simulink model "softMBD_old"  (R2025b)
settings: Solver=FixedStepAuto  StartTime=0.0  StopTime=10  FixedStep=0.005  RelTol=1e-3
values from neighbouring files (symbols this model uses):
  FPV_mass = 0.8    [Soft.m]
  g = 9.81    [Soft.m]
  ks = 0    [Soft.m]
  p_0 = 1013.25    [Soft.m]
  Q2Ts = forcetomotors()    [Soft.m]    (also in forcetomotors.m = inv(Ts2Q))
  takeOffDuration = 2    [Soft.m]
  Ts = 0.005    [Soft.m]
undefined symbols (not defined in the file or in its folder): DiscIntNeverNeededParam, kd_pq, kd_pr, kd_y, ki_pq, ki_pr, ki_t, ki_y, kp_pq, kp_pr, kp_y, pInitialization
libraries: simulink x35, discretizing x11, slpidlib x2, shared6dof x1, dynamicsLibrary x1, aerolibasang x1, aerolibnav x1
(part 17 of 20)

== system softMBD_old/FCS/Controller/roll_pitch_controller/PID Controller/Saturation Fdbk/Enabled ==
  In1 : Inport  SampleTime=SampleTime
  Saturation : Saturate  UpperLimit=UpperSaturationLimit  LowerLimit=LowerSaturationLimit  SampleTime=SampleTime  OutMin=SaturationOutMin  OutMax=SaturationOutMax
  Out1 : Outport  SampleTime=SampleTime
  wires:
  Saturation/1 -> Out1/1
  In1/1 -> Saturation/1

== system softMBD_old/FCS/Controller/roll_pitch_controller/PID Controller/Saturation Fdbk/External ==
  In1 : Inport  SampleTime=SampleTime
  Upper Limit : Inport  Port=2  SampleTime=SampleTime
  Lower Limit : Inport  Port=3  SampleTime=SampleTime
  Saturation Dynamic : simulink/Discontinuities/Saturation Dynamic  OutMin=SaturationOutMin  OutMax=SaturationOutMax  OutDataTypeStr=Inherit: Same as second input  OutDataType=fixdt(1, 16)  OutScaling=2^-10  DoSatur=off
  Out1 : Outport  SampleTime=SampleTime
  wires:
  Lower Limit/1 -> Saturation Dynamic/3
  Upper Limit/1 -> Saturation Dynamic/1
  Saturation Dynamic/1 -> Out1/1
  In1/1 -> Saturation Dynamic/2

== system softMBD_old/FCS/Controller/roll_pitch_controller/PID Controller/Saturation Fdbk/Passthrough ==
  In1 : Inport  SampleTime=SampleTime
  Out1 : Outport  SampleTime=SampleTime
  wires:
  In1/1 -> Out1/1

== system softMBD_old/FCS/Controller/roll_pitch_controller/PID Controller/Sum/Passthrough_I ==
  P : Inport  SampleTime=SampleTime
  I : Inport  Port=2  SampleTime=SampleTime
  Signal Specification : SignalSpecification  OutDataTypeStr=boolean  SampleTime=SampleTime
  Terminator : Terminator
  Out1 : Outport  SampleTime=SampleTime
  wires:
  Signal Specification/1 -> Terminator/1
  P/1 -> Signal Specification/1
  I/1 -> Out1/1

== system softMBD_old/FCS/Controller/roll_pitch_controller/PID Controller/Sum/Passthrough_P ==
  P : Inport  SampleTime=SampleTime
  Out1 : Outport  SampleTime=SampleTime
  wires:
  P/1 -> Out1/1

== system softMBD_old/FCS/Controller/roll_pitch_controller/PID Controller/Sum/Sum_PD ==
  P : Inport  SampleTime=SampleTime
  D : Inport  Port=2  SampleTime=SampleTime
  Sum : Sum  Inputs=|++  OutMin=SumOutMin  OutMax=SumOutMax
  Out1 : Outport  SampleTime=SampleTime
  wires:
  P/1 -> Sum/1
  D/1 -> Sum/2
  Sum/1 -> Out1/1

== system softMBD_old/FCS/Controller/roll_pitch_controller/PID Controller/Sum/Sum_PI ==
  P : Inport  SampleTime=SampleTime
  I : Inport  Port=2  SampleTime=SampleTime
  Sum : Sum  Inputs=|++  OutMin=SumOutMin  OutMax=SumOutMax
  Out1 : Outport  SampleTime=SampleTime
  wires:
  I/1 -> Sum/2
  P/1 -> Sum/1
  Sum/1 -> Out1/1

== system softMBD_old/FCS/Controller/roll_pitch_controller/PID Controller/Sum/Sum_PID ==
  P : Inport  SampleTime=SampleTime
  I : Inport  Port=2  SampleTime=SampleTime
  D : Inport  Port=3  SampleTime=SampleTime
  Sum : Sum  Inputs=+++  OutMin=SumOutMin  OutMax=SumOutMax
  Out1 : Outport  SampleTime=SampleTime
  wires:
  I/1 -> Sum/2
  P/1 -> Sum/1
  D/1 -> Sum/3
  Sum/1 -> Out1/1

== system softMBD_old/FCS/Controller/roll_pitch_controller/PID Controller/Sum Fdbk/Disabled ==
  fromP : Inport  SampleTime=SampleTime
  fromState : Inport  Port=2  SampleTime=SampleTime
  fromD : Inport  Port=3  SampleTime=SampleTime
  Signal Specification1 : SignalSpecification  DisableCoverage=on  OutDataTypeStr=boolean  SampleTime=SampleTime
  Terminator1 : Terminator
  Terminator2 : Terminator
  Terminator3 : Terminator
  wires:
  fromD/1 -> Terminator3/1
  fromState/1 -> Signal Specification1/1
  fromP/1 -> Terminator1/1
  Signal Specification1/1 -> Terminator2/1

== system softMBD_old/FCS/Controller/roll_pitch_controller/PID Controller/Sum Fdbk/Enabled ==
  fromP : Inport  SampleTime=SampleTime
  fromState : Inport  Port=2  SampleTime=SampleTime
  fromD : Inport  Port=3  SampleTime=SampleTime
  Sum Fdbk : Sum  DisableCoverage=on  Inputs=+++  OutMin=SumOutMin  OutMax=SumOutMax
  Out1 : Outport  SampleTime=SampleTime
  wires:
  fromP/1 -> Sum Fdbk/1
  fromState/1 -> Sum Fdbk/2
  fromD/1 -> Sum Fdbk/3
  Sum Fdbk/1 -> Out1/1

== system softMBD_old/FCS/Controller/roll_pitch_controller/PID Controller/Sum Fdbk/Passthrough ==
  fromState : Inport  SampleTime=SampleTime
  Out1 : Outport  SampleTime=SampleTime
  wires:
  fromState/1 -> Out1/1

== system softMBD_old/FCS/Controller/roll_pitch_controller/PID Controller/Tracking Mode/Disabled ==
  uout : Inport  SampleTime=SampleTime
  TR : Inport  Port=2  SampleTime=SampleTime
  Signal Specification1 : SignalSpecification  DisableCoverage=on  OutDataTypeStr=boolean  SampleTime=SampleTime
  Terminator1 : Terminator
  Terminator3 : Terminator
  wires:
  uout/1 -> Terminator3/1
  TR/1 -> Signal Specification1/1
  Signal Specification1/1 -> Terminator1/1

== system softMBD_old/FCS/Controller/roll_pitch_controller/PID Controller/Tracking Mode/Enabled ==
  uout : Inport  SampleTime=SampleTime
  TR : Inport  Port=2  SampleTime=SampleTime
  Kt : Gain  Gain=Kt  ParamMin=KtParamMin  ParamMax=KtParamMax  OutMin=KtOutMin  OutMax=KtOutMax
  SumI3 : Sum  Inputs=|-+  OutMin=SumI3OutMin  OutMax=SumI3OutMax
  Out1 : Outport  SampleTime=SampleTime
  wires:
  Kt/1 -> Out1/1
  SumI3/1 -> Kt/1
  TR/1 -> SumI3/2
  uout/1 -> SumI3/1

== system softMBD_old/FCS/Controller/roll_pitch_controller/PID Controller/Tracking Mode Sum/Passthrough ==
  fromIgain : Inport  SampleTime=SampleTime
  fromTR : Inport  Port=2  SampleTime=SampleTime
  Signal Specification : SignalSpecification  DisableCoverage=on  OutDataTypeStr=boolean  SampleTime=SampleTime
  Terminator : Terminator
  preInt : Outport
  wires:
  fromIgain/1 -> preInt/1
  fromTR/1 -> Signal Specification/1
  Signal Specification/1 -> Terminator/1

== system softMBD_old/FCS/Controller/roll_pitch_controller/PID Controller/Tracking Mode Sum/Tracking Mode ==
  fromIgain : Inport  SampleTime=SampleTime
  fromTR : Inport  Port=2  SampleTime=SampleTime
  SumI1 : Sum  Inputs=|++  OutMin=SumI1OutMin  OutMax=SumI1OutMax
  preInt : Outport
  wires:
  fromIgain/1 -> SumI1/1
  fromTR/1 -> SumI1/2
  SumI1/1 -> preInt/1

== system softMBD_old/FCS/Controller/roll_pitch_controller/PID Controller/Tsamp - Integral/Disabled ==
  U : Inport  SampleTime=SampleTime
  Ts : Inport  Port=2  SampleTime=SampleTime
  Terminator : Terminator
  Out1 : Outport  SampleTime=SampleTime
  wires:
  U/1 -> Out1/1
  Ts/1 -> Terminator/1

== system softMBD_old/FCS/Controller/roll_pitch_controller/PID Controller/Tsamp - Integral/External Ts ==
  U : Inport  SampleTime=SampleTime
  Ts : Inport  Port=2  SampleTime=SampleTime
  Uintegral*Ts Prod Out : Product  OutMin=UintegralTsProdOutMin  OutMax=UintegralTsProdOutMax  SampleTime=SampleTime
  Out1 : Outport  SampleTime=SampleTime
  wires:
  U/1 -> Uintegral*Ts Prod Out/1
  Uintegral*Ts Prod Out/1 -> Out1/1
  Ts/1 -> Uintegral*Ts Prod Out/2

== system softMBD_old/FCS/Controller/roll_pitch_controller/PID Controller/Tsamp - Integral/Passthrough ==
  U : Inport  SampleTime=SampleTime
  Ts : Inport  Port=2  SampleTime=SampleTime
  Terminator : Terminator
  Out1 : Outport  SampleTime=SampleTime
  wires:
  Ts/1 -> Terminator/1
  U/1 -> Out1/1

== system softMBD_old/FCS/Controller/roll_pitch_controller/PID Controller/Tsamp - Integral/TsSignalSpecification ==
  U : Inport  SampleTime=SampleTime
  Ts : Inport  Port=2  SampleTime=SampleTime
  Signal Specification : SignalSpecification  DisableCoverage=on  OutDataTypeStr=boolean  SampleTime=SampleTime
  Terminator : Terminator
  Out1 : Outport  SampleTime=SampleTime
  wires:
  U/1 -> Out1/1
  Ts/1 -> Signal Specification/1
  Signal Specification/1 -> Terminator/1

== system softMBD_old/FCS/Controller/roll_pitch_controller/PID Controller/Tsamp - Ngain/External Ts ==
  U : Inport  SampleTime=SampleTime
  Ts : Inport  Port=2  SampleTime=SampleTime
  Ungain*Ts Prod Out : Product  OutMin=UngainTsProdOutMin  OutMax=UngainTsProdOutMax  SampleTime=SampleTime
  Out1 : Outport  SampleTime=SampleTime
  wires:
  Ts/1 -> Ungain*Ts Prod Out/2
  Ungain*Ts Prod Out/1 -> Out1/1
  U/1 -> Ungain*Ts Prod Out/1

== system softMBD_old/FCS/Controller/roll_pitch_controller/PID Controller/Tsamp - Ngain/Passthrough ==
  U : Inport  SampleTime=SampleTime
  Ts : Inport  Port=2  SampleTime=SampleTime
  Terminator : Terminator
  Out1 : Outport  SampleTime=SampleTime
  wires:
  U/1 -> Out1/1
  Ts/1 -> Terminator/1

== system softMBD_old/FCS/Controller/roll_pitch_controller/PID Controller/postSat Signal/Feedback_Path ==
  feedback : Inport  SampleTime=SampleTime
  forward : Inport  Port=2  SampleTime=SampleTime
  Terminator1 : Terminator
  Out1 : Outport  SampleTime=SampleTime
  wires:
  feedback/1 -> Out1/1
  forward/1 -> Terminator1/1

== system softMBD_old/FCS/Controller/roll_pitch_controller/PID Controller/postSat Signal/Forward_Path ==
  feedback : Inport  SampleTime=SampleTime
  forward : Inport  Port=2  SampleTime=SampleTime
  Signal Specification1 : SignalSpecification  DisableCoverage=on  OutDataTypeStr=boolean  SampleTime=SampleTime
  Terminator1 : Terminator
  Out1 : Outport  SampleTime=SampleTime
  wires:
  forward/1 -> Out1/1
  feedback/1 -> Signal Specification1/1
  Signal Specification1/1 -> Terminator1/1

== system softMBD_old/FCS/Controller/roll_pitch_controller/PID Controller/preInt Signal/External PreInt ==
  preInt : Inport  SampleTime=SampleTime
  extAW : Inport  Port=2  SampleTime=SampleTime
  Terminator1 : Terminator
  Out1 : Outport  SampleTime=SampleTime
  wires:
  preInt/1 -> Terminator1/1
  extAW/1 -> Out1/1

== system softMBD_old/FCS/Controller/roll_pitch_controller/PID Controller/preInt Signal/Internal PreInt ==
  preInt : Inport  SampleTime=SampleTime
  extAW : Inport  Port=2  SampleTime=SampleTime
  Signal Specification1 : SignalSpecification  DisableCoverage=on  OutDataTypeStr=boolean  SampleTime=SampleTime
  Terminator1 : Terminator
  Out1 : Outport  SampleTime=SampleTime
  wires:
  Signal Specification1/1 -> Terminator1/1
  extAW/1 -> Signal Specification1/1
  preInt/1 -> Out1/1

== system softMBD_old/FCS/Controller/roll_pitch_controller/PID Controller/preSat Signal/Feedback_Path ==
  feedback : Inport  SampleTime=SampleTime
  forward : Inport  Port=2  SampleTime=SampleTime
  Terminator1 : Terminator
  Out1 : Outport  SampleTime=SampleTime
  wires:
  feedback/1 -> Out1/1
  forward/1 -> Terminator1/1

== system softMBD_old/FCS/Controller/roll_pitch_controller/PID Controller/preSat Signal/Forward_Path ==
  feedback : Inport  SampleTime=SampleTime
  forward : Inport  Port=2  SampleTime=SampleTime
  Signal Specification1 : SignalSpecification  DisableCoverage=on  OutDataTypeStr=boolean  SampleTime=SampleTime
  Terminator1 : Terminator
  Out1 : Outport  SampleTime=SampleTime
  wires:
  forward/1 -> Out1/1
  feedback/1 -> Signal Specification1/1
  Signal Specification1/1 -> Terminator1/1

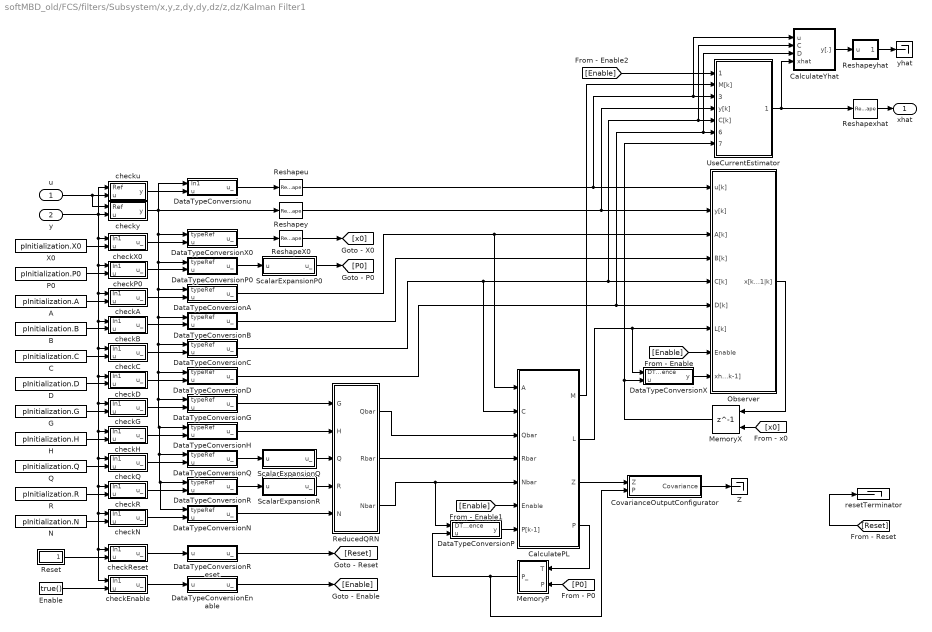
== system softMBD_old/FCS/filters/Subsystem/x,y,z,dy,dy,dz/z,dz/Kalman Filter1 ==
  u : Inport
  y : Inport  Port=2
  A : Constant  Value=pInitialization.A  VectorParams1D=off  OutDataTypeStr=Inherit: Inherit via back propagation
  B : Constant  Value=pInitialization.B  VectorParams1D=off  OutDataTypeStr=Inherit: Inherit via back propagation
  C : Constant  Value=pInitialization.C  VectorParams1D=off  OutDataTypeStr=Inherit: Inherit via back propagation
  CalculatePL : Subsystem  AncestorBlock=ctrlSharedLib/KalmanFilterUtilities/ConstantPL  mask(ctrlKalmanFilterConstantPL){}
  CalculateYhat : Subsystem  AncestorBlock=ctrlSharedLib/KalmanFilterUtilities/DontCalculateYhat  mask(ctrlKalmanFilterDontCalculateYhat){}
  CovarianceOutputConfigurator : Subsystem
  D : Constant  Value=pInitialization.D  VectorParams1D=off  OutDataTypeStr=Inherit: Inherit via back propagation
  DataTypeConversionA : Subsystem  AncestorBlock=ctrlSharedLib/Utilities/DataTypeDuplicateAndOutput  mask(ctrlDataTypeDuplicateAndOutput){}
  DataTypeConversionB : Subsystem  AncestorBlock=ctrlSharedLib/Utilities/DataTypeDuplicateAndOutput  mask(ctrlDataTypeDuplicateAndOutput){}
  DataTypeConversionC : Subsystem  AncestorBlock=ctrlSharedLib/Utilities/DataTypeDuplicateAndOutput  mask(ctrlDataTypeDuplicateAndOutput){}
  DataTypeConversionD : Subsystem  AncestorBlock=ctrlSharedLib/Utilities/DataTypeDuplicateAndOutput  mask(ctrlDataTypeDuplicateAndOutput){}
  DataTypeConversionEnable : Subsystem  AncestorBlock=ctrlSharedLib/Utilities/PassInputThrough
  DataTypeConversionG : Subsystem  AncestorBlock=ctrlSharedLib/Utilities/DataTypeDuplicateAndOutput  mask(ctrlDataTypeDuplicateAndOutput){}
  DataTypeConversionH : Subsystem  AncestorBlock=ctrlSharedLib/Utilities/DataTypeDuplicateAndOutput  mask(ctrlDataTypeDuplicateAndOutput){}
  DataTypeConversionN : Subsystem  AncestorBlock=ctrlSharedLib/Utilities/DataTypeDuplicateAndOutput  mask(ctrlDataTypeDuplicateAndOutput){}
  DataTypeConversionP : Subsystem  AncestorBlock=|  mask(Conversion Inherited){ConvertRealWorld=Real World Value, RndMeth=Floor, DoSatur=off}
      | simulink/Signal
      | Attributes/Data Type
      | Conversion
      | Inherited
      mask prompts: ConvertRealWorld "Simulink:masks:InputAndOutputToHaveEqual_MP"; RndMeth "Simulink:masks:IntegerRoundingMode_MP"; DoSatur "Simulink:masks:SaturateToMaxOrMinWhenOverflowsOccur_MP"
      mask help: Simulink:masks:ConversionInherited_MD
      mask init: same as softMBD_old/FCS/filters/Subsystem1/pitch_kalman/Kalman Filter1/DataTypeConversionP
      mask TypeOptions ConvertRealWorld: Simulink:masks:RealWorldValue | Simulink:masks:StoredInteger
      mask TypeOptions RndMeth: Simulink:masks:Ceiling | Simulink:masks:Convergent | Simulink:masks:Floor | Simulink:masks:Nearest | Simulink:masks:Round | Simulink:masks:Simplest | Simulink:masks:Zero
      mask Display:
      | port_label('Input',2,'u');
      | port_label('Output',1,'y');
      |     if(get_param(gcbh,'ConvertRealWorld') == "Stored Integer")
      |        disp('SI')
      |     else
      |        disp('Convert')
      |     end
  DataTypeConversionP0 : Subsystem  AncestorBlock=ctrlSharedLib/Utilities/DataTypeDuplicateAndOutput  mask(ctrlDataTypeDuplicateAndOutput){}
  DataTypeConversionQ : Subsystem  AncestorBlock=ctrlSharedLib/Utilities/DataTypeDuplicateAndOutput  mask(ctrlDataTypeDuplicateAndOutput){}
  DataTypeConversionR : Subsystem  AncestorBlock=ctrlSharedLib/Utilities/DataTypeDuplicateAndOutput  mask(ctrlDataTypeDuplicateAndOutput){}
  DataTypeConversionReset : Subsystem  AncestorBlock=ctrlSharedLib/Utilities/PassInputThrough
  DataTypeConversionX : Subsystem  AncestorBlock=|  mask(Conversion Inherited){ConvertRealWorld=Real World Value, RndMeth=Floor, DoSatur=off}
      | simulink/Signal
      | Attributes/Data Type
      | Conversion
      | Inherited
      mask prompts: ConvertRealWorld "Simulink:masks:InputAndOutputToHaveEqual_MP"; RndMeth "Simulink:masks:IntegerRoundingMode_MP"; DoSatur "Simulink:masks:SaturateToMaxOrMinWhenOverflowsOccur_MP"
      mask help: Simulink:masks:ConversionInherited_MD
      mask init: same as softMBD_old/FCS/filters/Subsystem1/pitch_kalman/Kalman Filter1/DataTypeConversionP
      mask TypeOptions ConvertRealWorld: Simulink:masks:RealWorldValue | Simulink:masks:StoredInteger
      mask TypeOptions RndMeth: Simulink:masks:Ceiling | Simulink:masks:Convergent | Simulink:masks:Floor | Simulink:masks:Nearest | Simulink:masks:Round | Simulink:masks:Simplest | Simulink:masks:Zero
      mask Display:
      | port_label('Input',2,'u');
      | port_label('Output',1,'y');
      |     if(get_param(gcbh,'ConvertRealWorld') == "Stored Integer")
      |        disp('SI')
      |     else
      |        disp('Convert')
      |     end
  DataTypeConversionX0 : Subsystem  AncestorBlock=ctrlSharedLib/Utilities/DataTypeDuplicateAndOutput  mask(ctrlDataTypeDuplicateAndOutput){}
  DataTypeConversionu : Subsystem  AncestorBlock=ctrlSharedLib/KalmanFilterUtilities/PassSecondInputThrough  mask(ctrlKalmanFilterPassSecondInputThrough){}
      mask Display:
      | port_label('Input',2,'u');
      | port_label('Output',1,'y');
  Enable : Constant  Value=true()  OutDataTypeStr=boolean
  G : Constant  Value=pInitialization.G  VectorParams1D=off  OutDataTypeStr=Inherit: Inherit via back propagation
  H : Constant  Value=pInitialization.H  VectorParams1D=off  OutDataTypeStr=Inherit: Inherit via back propagation
  MemoryP : Subsystem  AncestorBlock=ctrlSharedLib/KalmanFilterUtilities/MemoryP  mask(ctrlKalmanFilterNoMemoryP){}
      mask Display:
      | port_label('Input',2,'P');
      | port_label('Output',1,'P');
  MemoryX : Delay  DelayLength=1  InitialConditionSource=Input port  SampleTime=pInitialization.Ts
      settings: InputPortMap=u0,p4
  N : Constant  Value=pInitialization.N  VectorParams1D=off  OutDataTypeStr=Inherit: Inherit via back propagation
  Observer : Subsystem
  P0 : Constant  Value=pInitialization.P0  OutDataTypeStr=Inherit: Inherit via back propagation
  Q : Constant  Value=pInitialization.Q  VectorParams1D=off  OutDataTypeStr=Inherit: Inherit via back propagation
  R : Constant  Value=pInitialization.R  VectorParams1D=off  OutDataTypeStr=Inherit: Inherit via back propagation
  ReducedQRN : Subsystem  AncestorBlock=ctrlSharedLib/KalmanFilterUtilities/NoReducedQRN  mask(ctrlKalmanFilterNoReducedQRN){}
  Reset : Subsystem  AncestorBlock=ctrlSharedLib/Utilities/Ground  mask(ctrlSharedLibGround){OutDataTypeStr=boolean, Dimensions=1}
      mask prompts: OutDataTypeStr "Simulink:blkprm_prompts:UNIFIEDDATATYPE"; Dimensions "Simulink:blkprm_prompts:SigSpecDims"
      mask TypeOptions OutDataTypeStr: Signal Specification/OutDataTypeStr
      mask TypeOptions Dimensions: Signal Specification/Dimensions
      mask DialogControl OutDataTypeStr Prompt: Data type:
      mask DialogControl Dimensions Prompt: Dimensions (-1 for inherited):
  ReshapeX0 : Reshape
  Reshapeu : Reshape
  Reshapexhat : Reshape
  Reshapey : Reshape
  Reshapeyhat : Subsystem  AncestorBlock=ctrlSharedLib/Utilities/PassInputThrough
  ScalarExpansionP0 : Subsystem  AncestorBlock=ctrlSharedLib/Utilities/PassInputThrough
  ScalarExpansionQ : Subsystem  AncestorBlock=ctrlSharedLib/Utilities/PassInputThrough
  ScalarExpansionR : Subsystem  AncestorBlock=ctrlSharedLib/Utilities/PassInputThrough
  UseCurrentEstimator : Subsystem  AncestorBlock=ctrlSharedLib/KalmanFilterUtilities/UseCurrentEstimatorZeroD  mask(ctrlKalmanFilterUseCurrentEstimatorZeroD){}
  X0 : Constant  Value=pInitialization.X0  VectorParams1D=off  OutDataTypeStr=Inherit: Inherit via back propagation
  Z : Terminator
  checkA : Subsystem  AncestorBlock=ctrlSharedLib/KalmanFilterUtilities/PassSecondInputThrough  mask(ctrlKalmanFilterPassSecondInputThrough){}
      mask Display:
      | port_label('Input',2,'u');
      | port_label('Output',1,'y');
  checkB : Subsystem  AncestorBlock=ctrlSharedLib/KalmanFilterUtilities/PassSecondInputThrough  mask(ctrlKalmanFilterPassSecondInputThrough){}
      mask Display:
      | port_label('Input',2,'u');
      | port_label('Output',1,'y');
  checkC : Subsystem  AncestorBlock=ctrlSharedLib/KalmanFilterUtilities/PassSecondInputThrough  mask(ctrlKalmanFilterPassSecondInputThrough){}
      mask Display:
      | port_label('Input',2,'u');
      | port_label('Output',1,'y');
  checkD : Subsystem  AncestorBlock=ctrlSharedLib/KalmanFilterUtilities/PassSecondInputThrough  mask(ctrlKalmanFilterPassSecondInputThrough){}
      mask Display:
      | port_label('Input',2,'u');
      | port_label('Output',1,'y');
  checkEnable : Subsystem  AncestorBlock=ctrlSharedLib/KalmanFilterUtilities/PassSecondInputThrough  mask(ctrlKalmanFilterPassSecondInputThrough){}
      mask Display:
      | port_label('Input',2,'u');
      | port_label('Output',1,'y');
  checkG : Subsystem  AncestorBlock=ctrlSharedLib/KalmanFilterUtilities/PassSecondInputThrough  mask(ctrlKalmanFilterPassSecondInputThrough){}
      mask Display:
      | port_label('Input',2,'u');
      | port_label('Output',1,'y');
  checkH : Subsystem  AncestorBlock=ctrlSharedLib/KalmanFilterUtilities/PassSecondInputThrough  mask(ctrlKalmanFilterPassSecondInputThrough){}
      mask Display:
      | port_label('Input',2,'u');
      | port_label('Output',1,'y');
  checkN : Subsystem  AncestorBlock=ctrlSharedLib/KalmanFilterUtilities/PassSecondInputThrough  mask(ctrlKalmanFilterPassSecondInputThrough){}
      mask Display:
      | port_label('Input',2,'u');
      | port_label('Output',1,'y');
  checkP0 : Subsystem  AncestorBlock=ctrlSharedLib/KalmanFilterUtilities/PassSecondInputThrough  mask(ctrlKalmanFilterPassSecondInputThrough){}
      mask Display:
      | port_label('Input',2,'u');
      | port_label('Output',1,'y');
  checkQ : Subsystem  AncestorBlock=ctrlSharedLib/KalmanFilterUtilities/PassSecondInputThrough  mask(ctrlKalmanFilterPassSecondInputThrough){}
      mask Display:
      | port_label('Input',2,'u');
      | port_label('Output',1,'y');
  checkR : Subsystem  AncestorBlock=ctrlSharedLib/KalmanFilterUtilities/PassSecondInputThrough  mask(ctrlKalmanFilterPassSecondInputThrough){}
      mask Display:
      | port_label('Input',2,'u');
      | port_label('Output',1,'y');
  checkReset : Subsystem  AncestorBlock=ctrlSharedLib/KalmanFilterUtilities/PassSecondInputThrough  mask(ctrlKalmanFilterPassSecondInputThrough){}
      mask Display:
      | port_label('Input',2,'u');
      | port_label('Output',1,'y');
  checkX0 : Subsystem  AncestorBlock=ctrlSharedLib/KalmanFilterUtilities/PassSecondInputThrough  mask(ctrlKalmanFilterPassSecondInputThrough){}
      mask Display:
      | port_label('Input',2,'u');
      | port_label('Output',1,'y');
  checku : Subsystem  AncestorBlock=ctrlSharedLib/KalmanFilterUtilities/checkSignals  mask(ctrlKalmanFilterCheckSignals){Ts=pInitialization.Ts, Ns=pInitialization.Ns, Nu=pInitialization.Nu, Nw=pInitialization.Nw, Ny=pInitialization.Ny}
      mask prompts: Ts "Sample time:"; Ns "Number of states:"; Nu "Number of inputs:"; Nw "Number of process noise inputs:"; Ny "Number of outputs:"
      mask init: same as softMBD_old/FCS/filters/Subsystem1/pitch_kalman/Kalman Filter1/checku
      mask DialogControl ParametersContainer Prompt: Parameters
  checky : Subsystem  AncestorBlock=ctrlSharedLib/KalmanFilterUtilities/checkSignals  mask(ctrlKalmanFilterCheckSignals){Ts=pInitialization.Ts, Ns=pInitialization.Ns, Nu=pInitialization.Nu, Nw=pInitialization.Nw, Ny=pInitialization.Ny}
      mask prompts: Ts "Sample time:"; Ns "Number of states:"; Nu "Number of inputs:"; Nw "Number of process noise inputs:"; Ny "Number of outputs:"
      mask init: same as softMBD_old/FCS/filters/Subsystem1/pitch_kalman/Kalman Filter1/checku
      mask DialogControl ParametersContainer Prompt: Parameters
  resetTerminator : Terminator
  yhat : Terminator
  xhat : Outport  VectorParamsAs1DForOutWhenUnconnected=off
  wires:
  [Reset] -> resetTerminator/1
  CalculatePL/3(Z) -> CovarianceOutputConfigurator/1(Z)
  Reshapexhat/1 -> xhat/1
  Reshapeyhat/1(u_) -> yhat/1
  UseCurrentEstimator/1(xhat[k|k]) -> Reshapexhat/1, CalculateYhat/4(xhat)
  checku/1(y) -> DataTypeConversionu/2(u)
  DataTypeConversionu/1(u_) -> Reshapeu/1
  CovarianceOutputConfigurator/1(Covariance) -> Z/1
  DataTypeConversionC/1(u_) -> Observer/5(C[k]), UseCurrentEstimator/5(C[k]), CalculateYhat/2(C), CalculatePL/2(C)
  ScalarExpansionR/1(u_) -> ReducedQRN/4(R)
  ScalarExpansionQ/1(u_) -> ReducedQRN/3(Q)
  ScalarExpansionP0/1(u_) -> [P0]
  CalculatePL/4(P) -> MemoryP/1(T)
  DataTypeConversionReset/1(u_) -> [Reset]
  checkReset/1(u_) -> DataTypeConversionReset/1(u)
  checky/1(y) -> DataTypeConversionX0/1(typeRef), DataTypeConversionP0/1(typeRef), DataTypeConversionC/1(typeRef), DataTypeConversionD/1(typeRef), DataTypeConversionG/1(typeRef), DataTypeConversionH/1(typeRef), DataTypeConversionQ/1(typeRef), DataTypeConversionR/1(typeRef), DataTypeConversionN/1(typeRef), DataTypeConversionB/1(typeRef), DataTypeConversionA/1(typeRef), Reshapey/1, DataTypeConversionu/1(In1)
  ReshapeX0/1 -> [x0]
  MemoryP/1(P_) -> DataTypeConversionP/2(u), CovarianceOutputConfigurator/2(P)
  [P0] -> MemoryP/2(P)
  CalculateYhat/1(y[.]) -> Reshapeyhat/1(u)
  [Enable] -> UseCurrentEstimator/1(Enable[k])
  CalculatePL/1(M) -> UseCurrentEstimator/2(M[k])
  CalculatePL/2(L) -> Observer/7(L[k]), DataTypeConversionX/1(DTS reference)
  Reshapey/1 -> Observer/2(y[k]), UseCurrentEstimator/4(y[k])
  Reshapeu/1 -> Observer/1(u[k]), UseCurrentEstimator/3(u (unused)), CalculateYhat/1(u)
  y/1 -> checky/2(u), checku/1(Ref), checkX0/1(In1), checkP0/1(In1), checkA/1(In1), checkB/1(In1), checkC/1(In1), checkD/1(In1), checkG/1(In1), checkH/1(In1), checkQ/1(In1), checkR/1(In1), checkN/1(In1), checkReset/1(In1), checkEnable/1(In1)
  u/1 -> checku/2(u), checky/1(Ref)
  DataTypeConversionP/1(y) -> CalculatePL/7(P[k-1])
  [Enable] -> Observer/8(Enable)
  DataTypeConversionX/1(y) -> Observer/9(xhat[k|k-1])
  DataTypeConversionX0/1(u_) -> ReshapeX0/1
  [x0] -> MemoryX/2
  X0/1 -> checkX0/2(u)
  DataTypeConversionD/1(u_) -> Observer/6(D[k]), UseCurrentEstimator/6(D (unused)), CalculateYhat/3(D)
  DataTypeConversionB/1(u_) -> Observer/4(B[k])
  DataTypeConversionA/1(u_) -> Observer/3(A[k]), CalculatePL/1(A)
  checkB/1(u_) -> DataTypeConversionB/2(u)
  B/1 -> checkB/2(u)
  ReducedQRN/3(Nbar) -> CalculatePL/5(Nbar), DataTypeConversionP/1(DTS reference)
  ReducedQRN/2(Rbar) -> CalculatePL/4(Rbar)
  ReducedQRN/1(Qbar) -> CalculatePL/3(Qbar)
  checkA/1(u_) -> DataTypeConversionA/2(u)
  A/1 -> checkA/2(u)
  [Enable] -> CalculatePL/6(Enable)
  Observer/1(x[k+1|k]) -> MemoryX/1
  DataTypeConversionEnable/1(u_) -> [Enable]
  checkEnable/1(u_) -> DataTypeConversionEnable/1(u)
  Enable/1 -> checkEnable/2(u)
  DataTypeConversionP0/1(u_) -> ScalarExpansionP0/1(u)
  Reset/1(Out) -> checkReset/2(u)
  DataTypeConversionN/1(u_) -> ReducedQRN/5(N)
  checkN/1(u_) -> DataTypeConversionN/2(u)
  checkR/1(u_) -> DataTypeConversionR/2(u)
  DataTypeConversionR/1(u_) -> ScalarExpansionR/1(u)
  checkQ/1(u_) -> DataTypeConversionQ/2(u)
  DataTypeConversionQ/1(u_) -> ScalarExpansionQ/1(u)
  DataTypeConversionH/1(u_) -> ReducedQRN/2(H)
  checkH/1(u_) -> DataTypeConversionH/2(u)
  DataTypeConversionG/1(u_) -> ReducedQRN/1(G)
  checkG/1(u_) -> DataTypeConversionG/2(u)
  checkD/1(u_) -> DataTypeConversionD/2(u)
  checkC/1(u_) -> DataTypeConversionC/2(u)
  checkP0/1(u_) -> DataTypeConversionP0/2(u)
  checkX0/1(u_) -> DataTypeConversionX0/2(u)
  MemoryX/1 -> DataTypeConversionX/2(u), UseCurrentEstimator/7(xhat[k|k-1])
  N/1 -> checkN/2(u)
  R/1 -> checkR/2(u)
  Q/1 -> checkQ/2(u)
  H/1 -> checkH/2(u)
  G/1 -> checkG/2(u)
  D/1 -> checkD/2(u)
  P0/1 -> checkP0/2(u)
  C/1 -> checkC/2(u)

== system softMBD_old/FCS/filters/Subsystem1/pitch_kalman/Kalman Filter1/CalculatePL ==
  A : Inport
  C : Inport  Port=2
  Qbar : Inport  Port=3
  Rbar : Inport  Port=4
  Nbar : Inport  Port=5
  Enable : Inport  Port=6
  P[k-1] : Inport  Port=7
  CovarianceZ : Constant  Value=pInitialization.Z
  DataTypeConversionL : Subsystem  AncestorBlock=|  mask(Conversion Inherited){ConvertRealWorld=Real World Value, RndMeth=Floor, DoSatur=off}
      | simulink/Signal
      | Attributes/Data Type
      | Conversion
      | Inherited
      mask prompts: ConvertRealWorld "Simulink:masks:InputAndOutputToHaveEqual_MP"; RndMeth "Simulink:masks:IntegerRoundingMode_MP"; DoSatur "Simulink:masks:SaturateToMaxOrMinWhenOverflowsOccur_MP"
      mask help: Simulink:masks:ConversionInherited_MD
      mask init: same as softMBD_old/FCS/filters/Subsystem1/pitch_kalman/Kalman Filter1/DataTypeConversionP
      mask TypeOptions ConvertRealWorld: Simulink:masks:RealWorldValue | Simulink:masks:StoredInteger
      mask TypeOptions RndMeth: Simulink:masks:Ceiling | Simulink:masks:Convergent | Simulink:masks:Floor | Simulink:masks:Nearest | Simulink:masks:Round | Simulink:masks:Simplest | Simulink:masks:Zero
      mask Display:
      | port_label('Input',2,'u');
      | port_label('Output',1,'y');
      |     if(get_param(gcbh,'ConvertRealWorld') == "Stored Integer")
      |        disp('SI')
      |     else
      |        disp('Convert')
      |     end
  DataTypeConversionM : Subsystem  AncestorBlock=|  mask(Conversion Inherited){ConvertRealWorld=Real World Value, RndMeth=Floor, DoSatur=off}
      | simulink/Signal
      | Attributes/Data Type
      | Conversion
      | Inherited
      mask prompts: ConvertRealWorld "Simulink:masks:InputAndOutputToHaveEqual_MP"; RndMeth "Simulink:masks:IntegerRoundingMode_MP"; DoSatur "Simulink:masks:SaturateToMaxOrMinWhenOverflowsOccur_MP"
      mask help: Simulink:masks:ConversionInherited_MD
      mask init: same as softMBD_old/FCS/filters/Subsystem1/pitch_kalman/Kalman Filter1/DataTypeConversionP
      mask TypeOptions ConvertRealWorld: Simulink:masks:RealWorldValue | Simulink:masks:StoredInteger
      mask TypeOptions RndMeth: Simulink:masks:Ceiling | Simulink:masks:Convergent | Simulink:masks:Floor | Simulink:masks:Nearest | Simulink:masks:Round | Simulink:masks:Simplest | Simulink:masks:Zero
      mask Display:
      | port_label('Input',2,'u');
      | port_label('Output',1,'y');
      |     if(get_param(gcbh,'ConvertRealWorld') == "Stored Integer")
      |        disp('SI')
      |     else
      |        disp('Convert')
      |     end
  DataTypeConversionP : Subsystem  AncestorBlock=|  mask(Conversion Inherited){ConvertRealWorld=Real World Value, RndMeth=Floor, DoSatur=off}
      | simulink/Signal
      | Attributes/Data Type
      | Conversion
      | Inherited
      mask prompts: ConvertRealWorld "Simulink:masks:InputAndOutputToHaveEqual_MP"; RndMeth "Simulink:masks:IntegerRoundingMode_MP"; DoSatur "Simulink:masks:SaturateToMaxOrMinWhenOverflowsOccur_MP"
      mask help: Simulink:masks:ConversionInherited_MD
      mask init: same as softMBD_old/FCS/filters/Subsystem1/pitch_kalman/Kalman Filter1/DataTypeConversionP
      mask TypeOptions ConvertRealWorld: Simulink:masks:RealWorldValue | Simulink:masks:StoredInteger
      mask TypeOptions RndMeth: Simulink:masks:Ceiling | Simulink:masks:Convergent | Simulink:masks:Floor | Simulink:masks:Nearest | Simulink:masks:Round | Simulink:masks:Simplest | Simulink:masks:Zero
      mask Display:
      | port_label('Input',2,'u');
      | port_label('Output',1,'y');
      |     if(get_param(gcbh,'ConvertRealWorld') == "Stored Integer")
      |        disp('SI')
      |     else
      |        disp('Convert')
      |     end
  DataTypeConversionZ : Subsystem  AncestorBlock=|  mask(Conversion Inherited){ConvertRealWorld=Real World Value, RndMeth=Floor, DoSatur=off}
      | simulink/Signal
      | Attributes/Data Type
      | Conversion
      | Inherited
      mask prompts: ConvertRealWorld "Simulink:masks:InputAndOutputToHaveEqual_MP"; RndMeth "Simulink:masks:IntegerRoundingMode_MP"; DoSatur "Simulink:masks:SaturateToMaxOrMinWhenOverflowsOccur_MP"
      mask help: Simulink:masks:ConversionInherited_MD
      mask init: same as softMBD_old/FCS/filters/Subsystem1/pitch_kalman/Kalman Filter1/DataTypeConversionP
      mask TypeOptions ConvertRealWorld: Simulink:masks:RealWorldValue | Simulink:masks:StoredInteger
      mask TypeOptions RndMeth: Simulink:masks:Ceiling | Simulink:masks:Convergent | Simulink:masks:Floor | Simulink:masks:Nearest | Simulink:masks:Round | Simulink:masks:Simplest | Simulink:masks:Zero
      mask Display:
      | port_label('Input',2,'u');
      | port_label('Output',1,'y');
      |     if(get_param(gcbh,'ConvertRealWorld') == "Stored Integer")
      |        disp('SI')
      |     else
      |        disp('Convert')
      |     end
  Ground : Subsystem  AncestorBlock=ctrlSharedLib/Utilities/Ground  mask(ctrlSharedLibGround){OutDataTypeStr=single, Dimensions=1}
      mask prompts: OutDataTypeStr "Simulink:blkprm_prompts:UNIFIEDDATATYPE"; Dimensions "Simulink:blkprm_prompts:SigSpecDims"
      mask TypeOptions OutDataTypeStr: Signal Specification/OutDataTypeStr
      mask TypeOptions Dimensions: Signal Specification/Dimensions
      mask DialogControl OutDataTypeStr Prompt: Data type:
      mask DialogControl Dimensions Prompt: Dimensions (-1 for inherited):
  KalmanGainL : Constant  Value=pInitialization.L
  KalmanGainM : Constant  Value=pInitialization.M
  Terminator{,2,4..8} (7 alike) : Terminator
  M : Outport  VectorParamsAs1DForOutWhenUnconnected=off
  L : Outport  Port=2  VectorParamsAs1DForOutWhenUnconnected=off
  Z : Outport  Port=3  VectorParamsAs1DForOutWhenUnconnected=off
  P : Outport  Port=4  VectorParamsAs1DForOutWhenUnconnected=off
  wires:
  DataTypeConversionP/1(y) -> P/1
  CovarianceZ/1 -> DataTypeConversionZ/2(u)
  DataTypeConversionZ/1(y) -> Z/1
  Ground/1(Out) -> DataTypeConversionP/2(u)
  DataTypeConversionM/1(y) -> M/1
  KalmanGainM/1 -> DataTypeConversionM/2(u)
  P[k-1]/1 -> Terminator8/1
  Enable/1 -> Terminator7/1
  KalmanGainL/1 -> DataTypeConversionL/2(u)
  DataTypeConversionL/1(y) -> L/1
  Nbar/1 -> Terminator6/1
  Rbar/1 -> Terminator5/1
  Qbar/1 -> Terminator4/1
  C/1 -> Terminator2/1, DataTypeConversionL/1(DTS reference), DataTypeConversionM/1(DTS reference), DataTypeConversionZ/1(DTS reference), DataTypeConversionP/1(DTS reference)
  A/1 -> Terminator/1

== system softMBD_old/FCS/filters/Subsystem1/pitch_kalman/Kalman Filter1/CalculateYhat ==
  u : Inport  SampleTime=pInitialization.Ts
  C : Inport  Port=2  SampleTime=pInitialization.Ts
  D : Inport  Port=3  SampleTime=pInitialization.Ts
  xhat : Inport  Port=4  SampleTime=pInitialization.Ts
  Ground : Subsystem  AncestorBlock=ctrlSharedLib/Utilities/Ground  mask(ctrlSharedLibGround){OutDataTypeStr=single, Dimensions=1}
      mask prompts: OutDataTypeStr "Simulink:blkprm_prompts:UNIFIEDDATATYPE"; Dimensions "Simulink:blkprm_prompts:SigSpecDims"
      mask TypeOptions OutDataTypeStr: Signal Specification/OutDataTypeStr
      mask TypeOptions Dimensions: Signal Specification/Dimensions
      mask DialogControl OutDataTypeStr Prompt: Data type:
      mask DialogControl Dimensions Prompt: Dimensions (-1 for inherited):
  TerminatorC : Terminator
  TerminatorD : Terminator
  Terminatoru : Terminator
  Terminatorxhat : Terminator
  y[.] : Outport  VectorParamsAs1DForOutWhenUnconnected=off
  wires:
  Ground/1(Out) -> y[.]/1
  u/1 -> Terminatoru/1
  D/1 -> TerminatorD/1
  xhat/1 -> Terminatorxhat/1
  C/1 -> TerminatorC/1

== system softMBD_old/FCS/filters/Subsystem1/pitch_kalman/Kalman Filter1/CovarianceOutputConfigurator ==
  Z : Inport
  P : Inport  Port=2
  TerminatorP : Terminator
  TerminatorZ : Terminator
  decideOutput : Subsystem  mask(outputZorP){}
  Covariance : Outport  VectorParamsAs1DForOutWhenUnconnected=off
  wires:
  decideOutput/1(P) -> Covariance/1
  P/1 -> TerminatorP/1
  Z/1 -> TerminatorZ/1, decideOutput/1(Z)

== system softMBD_old/FCS/filters/Subsystem1/pitch_kalman/Kalman Filter1/DataTypeConversionA ==
  typeRef : Inport
  u : Inport  Port=2
  Data Type Duplicate : DataTypeDuplicate
  u_ : Outport  VectorParamsAs1DForOutWhenUnconnected=off
  wires:
  typeRef/1 -> Data Type Duplicate/1
  u/1 -> Data Type Duplicate/2, u_/1

== system softMBD_old/FCS/filters/Subsystem1/pitch_kalman/Kalman Filter1/DataTypeConversionB ==
  typeRef : Inport
  u : Inport  Port=2
  Data Type Duplicate : DataTypeDuplicate
  u_ : Outport  VectorParamsAs1DForOutWhenUnconnected=off
  wires:
  typeRef/1 -> Data Type Duplicate/1
  u/1 -> Data Type Duplicate/2, u_/1

== system softMBD_old/FCS/filters/Subsystem1/pitch_kalman/Kalman Filter1/DataTypeConversionC ==
  typeRef : Inport
  u : Inport  Port=2
  Data Type Duplicate : DataTypeDuplicate
  u_ : Outport  VectorParamsAs1DForOutWhenUnconnected=off
  wires:
  typeRef/1 -> Data Type Duplicate/1
  u/1 -> Data Type Duplicate/2, u_/1

== system softMBD_old/FCS/filters/Subsystem1/pitch_kalman/Kalman Filter1/DataTypeConversionD ==
  typeRef : Inport
  u : Inport  Port=2
  Data Type Duplicate : DataTypeDuplicate
  u_ : Outport  VectorParamsAs1DForOutWhenUnconnected=off
  wires:
  typeRef/1 -> Data Type Duplicate/1
  u/1 -> Data Type Duplicate/2, u_/1

== system softMBD_old/FCS/filters/Subsystem1/pitch_kalman/Kalman Filter1/DataTypeConversionEnable ==
  u : Inport
  u_ : Outport  VectorParamsAs1DForOutWhenUnconnected=off
  wires:
  u/1 -> u_/1

== system softMBD_old/FCS/filters/Subsystem1/pitch_kalman/Kalman Filter1/DataTypeConversionG ==
  typeRef : Inport
  u : Inport  Port=2
  Data Type Duplicate : DataTypeDuplicate
  u_ : Outport  VectorParamsAs1DForOutWhenUnconnected=off
  wires:
  typeRef/1 -> Data Type Duplicate/1
  u/1 -> Data Type Duplicate/2, u_/1

== system softMBD_old/FCS/filters/Subsystem1/pitch_kalman/Kalman Filter1/DataTypeConversionH ==
  typeRef : Inport
  u : Inport  Port=2
  Data Type Duplicate : DataTypeDuplicate
  u_ : Outport  VectorParamsAs1DForOutWhenUnconnected=off
  wires:
  typeRef/1 -> Data Type Duplicate/1
  u/1 -> Data Type Duplicate/2, u_/1

== system softMBD_old/FCS/filters/Subsystem1/pitch_kalman/Kalman Filter1/DataTypeConversionN ==
  typeRef : Inport
  u : Inport  Port=2
  Data Type Duplicate : DataTypeDuplicate
  u_ : Outport  VectorParamsAs1DForOutWhenUnconnected=off
  wires:
  typeRef/1 -> Data Type Duplicate/1
  u/1 -> Data Type Duplicate/2, u_/1

== system softMBD_old/FCS/filters/Subsystem1/pitch_kalman/Kalman Filter1/DataTypeConversionP ==
  DTS reference : Inport
  u : Inport  Port=2
  Conversion : DataTypeConversion  SaturateOnIntegerOverflow=off  RndMeth=Floor  LockScale=on
  Data Type Duplicate : DataTypeDuplicate  DisableCoverage=on
  y : Outport
  wires:
  Conversion/1 -> Data Type Duplicate/2, y/1
  DTS reference/1 -> Data Type Duplicate/1
  u/1 -> Conversion/1

== system softMBD_old/FCS/filters/Subsystem1/pitch_kalman/Kalman Filter1/DataTypeConversionP0 ==
  typeRef : Inport
  u : Inport  Port=2
  Data Type Duplicate : DataTypeDuplicate
  u_ : Outport  VectorParamsAs1DForOutWhenUnconnected=off
  wires:
  typeRef/1 -> Data Type Duplicate/1
  u/1 -> Data Type Duplicate/2, u_/1

== system softMBD_old/FCS/filters/Subsystem1/pitch_kalman/Kalman Filter1/DataTypeConversionQ ==
  typeRef : Inport
  u : Inport  Port=2
  Data Type Duplicate : DataTypeDuplicate
  u_ : Outport  VectorParamsAs1DForOutWhenUnconnected=off
  wires:
  typeRef/1 -> Data Type Duplicate/1
  u/1 -> Data Type Duplicate/2, u_/1

== system softMBD_old/FCS/filters/Subsystem1/pitch_kalman/Kalman Filter1/DataTypeConversionR ==
  typeRef : Inport
  u : Inport  Port=2
  Data Type Duplicate : DataTypeDuplicate
  u_ : Outport  VectorParamsAs1DForOutWhenUnconnected=off
  wires:
  typeRef/1 -> Data Type Duplicate/1
  u/1 -> Data Type Duplicate/2, u_/1

== system softMBD_old/FCS/filters/Subsystem1/pitch_kalman/Kalman Filter1/DataTypeConversionReset ==
  u : Inport
  u_ : Outport  VectorParamsAs1DForOutWhenUnconnected=off
  wires:
  u/1 -> u_/1

== system softMBD_old/FCS/filters/Subsystem1/pitch_kalman/Kalman Filter1/DataTypeConversionX ==
  DTS reference : Inport
  u : Inport  Port=2
  Conversion : DataTypeConversion  SaturateOnIntegerOverflow=off  RndMeth=Floor  LockScale=on
  Data Type Duplicate : DataTypeDuplicate  DisableCoverage=on
  y : Outport
  wires:
  Conversion/1 -> Data Type Duplicate/2, y/1
  DTS reference/1 -> Data Type Duplicate/1
  u/1 -> Conversion/1

== system softMBD_old/FCS/filters/Subsystem1/pitch_kalman/Kalman Filter1/DataTypeConversionX0 ==
  typeRef : Inport
  u : Inport  Port=2
  Data Type Duplicate : DataTypeDuplicate
  u_ : Outport  VectorParamsAs1DForOutWhenUnconnected=off
  wires:
  typeRef/1 -> Data Type Duplicate/1
  u/1 -> Data Type Duplicate/2, u_/1

== system softMBD_old/FCS/filters/Subsystem1/pitch_kalman/Kalman Filter1/DataTypeConversionu ==
  In1 : Inport
  u : Inport  Port=2
  Terminator : Terminator
  u_ : Outport  VectorParamsAs1DForOutWhenUnconnected=off
  wires:
  In1/1 -> Terminator/1
  u/1 -> u_/1

== system softMBD_old/FCS/filters/Subsystem1/pitch_kalman/Kalman Filter1/MemoryP ==
  T : Inport
  P : Inport  Port=2
  Terminator : Terminator
  P_ : Outport  VectorParamsAs1DForOutWhenUnconnected=off
  wires:
  T/1 -> Terminator/1
  P/1 -> P_/1

== system softMBD_old/FCS/filters/Subsystem1/pitch_kalman/Kalman Filter1/Observer ==
  note: A*xhat+B*u+L*(yMeas-yHat)
      | or
      | A*xhat+B*u
  u[k] : Inport  SampleTime=pInitialization.Ts
  y[k] : Inport  Port=2  SampleTime=pInitialization.Ts
  A[k] : Inport  Port=3  SampleTime=pInitialization.Ts
  B[k] : Inport  Port=4  SampleTime=pInitialization.Ts
  C[k] : Inport  Port=5  SampleTime=pInitialization.Ts
  D[k] : Inport  Port=6  SampleTime=pInitialization.Ts
  L[k] : Inport  Port=7  SampleTime=pInitialization.Ts
  Enable : Inport  Port=8  SampleTime=pInitialization.Ts
  xhat[k|k-1] : Inport  Port=9  SampleTime=pInitialization.Ts
  A[k]*xhat[k|k-1] : Product  Multiplication=Matrix(*)
  Add : Sum  Inputs=+++
  B[k]*u[k] : Product  Multiplication=Matrix(*)
  MeasurementUpdate : Subsystem  TreatAsAtomicUnit=on
  Reshape : Reshape
  x[k+1|k] : Outport  SampleTime=pInitialization.Ts  VectorParamsAs1DForOutWhenUnconnected=off
  wires:
  D[k]/1 -> MeasurementUpdate/5(D[k])
  Reshape/1 -> x[k+1|k]/1
  y[k]/1 -> MeasurementUpdate/2(y[k])
  C[k]/1 -> MeasurementUpdate/3(C[k])
  MeasurementUpdate/1(L*(y[k]-yhat[k|k-1])) -> Add/3
  A[k]/1 -> A[k]*xhat[k|k-1]/1
  xhat[k|k-1]/1 -> A[k]*xhat[k|k-1]/2, MeasurementUpdate/4(xhat[k|k-1])
  B[k]/1 -> B[k]*u[k]/1
  L[k]/1 -> MeasurementUpdate/1(L[k])
  A[k]*xhat[k|k-1]/1 -> Add/2
  u[k]/1 -> B[k]*u[k]/2, MeasurementUpdate/6(u[k])
  Add/1 -> Reshape/1
  B[k]*u[k]/1 -> Add/1
  Enable/1 -> MeasurementUpdate/Enable

== system softMBD_old/FCS/filters/Subsystem1/pitch_kalman/Kalman Filter1/ReducedQRN ==
  G : Inport  SampleTime=pInitialization.Ts
  H : Inport  Port=2  SampleTime=pInitialization.Ts
  Q : Inport  Port=3  SampleTime=pInitialization.Ts
  R : Inport  Port=4  SampleTime=pInitialization.Ts
  N : Inport  Port=5  SampleTime=pInitialization.Ts
  Ground : Subsystem  AncestorBlock=ctrlSharedLib/Utilities/Ground  mask(ctrlSharedLibGround){OutDataTypeStr=single, Dimensions=1}
      mask prompts: OutDataTypeStr "Simulink:blkprm_prompts:UNIFIEDDATATYPE"; Dimensions "Simulink:blkprm_prompts:SigSpecDims"
      mask TypeOptions OutDataTypeStr: Signal Specification/OutDataTypeStr
      mask TypeOptions Dimensions: Signal Specification/Dimensions
      mask DialogControl OutDataTypeStr Prompt: Data type:
      mask DialogControl Dimensions Prompt: Dimensions (-1 for inherited):
  Terminator{,1..4} (5 alike) : Terminator
  Qbar : Outport  SampleTime=pInitialization.Ts  VectorParamsAs1DForOutWhenUnconnected=off
  Rbar : Outport  Port=2  SampleTime=pInitialization.Ts  VectorParamsAs1DForOutWhenUnconnected=off
  Nbar : Outport  Port=3  SampleTime=pInitialization.Ts  VectorParamsAs1DForOutWhenUnconnected=off
  wires:
  Ground/1(Out) -> Rbar/1, Nbar/1, Qbar/1
  N/1 -> Terminator4/1
  R/1 -> Terminator3/1
  Q/1 -> Terminator2/1
  H/1 -> Terminator1/1
  G/1 -> Terminator/1

== system softMBD_old/FCS/filters/Subsystem1/pitch_kalman/Kalman Filter1/Reset ==
  note: Specification is to avoid underspecified data type warnings in the code generation process
  Ground : Ground
  Signal Specification : SignalSpecification  OutDataTypeStr=boolean  Dimensions=1
  Out : Outport  VectorParamsAs1DForOutWhenUnconnected=off
  wires:
  Signal Specification/1 -> Out/1
  Ground/1 -> Signal Specification/1

== system softMBD_old/FCS/filters/Subsystem1/pitch_kalman/Kalman Filter1/Reshapeyhat ==
  u : Inport
  u_ : Outport  VectorParamsAs1DForOutWhenUnconnected=off
  wires:
  u/1 -> u_/1

== system softMBD_old/FCS/filters/Subsystem1/pitch_kalman/Kalman Filter1/ScalarExpansionP0 ==
  u : Inport
  u_ : Outport  VectorParamsAs1DForOutWhenUnconnected=off
  wires:
  u/1 -> u_/1

== system softMBD_old/FCS/filters/Subsystem1/pitch_kalman/Kalman Filter1/ScalarExpansionQ ==
  u : Inport
  u_ : Outport  VectorParamsAs1DForOutWhenUnconnected=off
  wires:
  u/1 -> u_/1

== system softMBD_old/FCS/filters/Subsystem1/pitch_kalman/Kalman Filter1/ScalarExpansionR ==
  u : Inport
  u_ : Outport  VectorParamsAs1DForOutWhenUnconnected=off
  wires:
  u/1 -> u_/1

== system softMBD_old/FCS/filters/Subsystem1/pitch_kalman/Kalman Filter1/UseCurrentEstimator ==
  note: System model has D=0
      | Break connection, avoid fictitious algebraic loop
  Enable[k] : Inport  SampleTime=pInitialization.Ts
  M[k] : Inport  Port=2  SampleTime=pInitialization.Ts
  u (unused) : Inport  Port=3  SampleTime=pInitialization.Ts
  y[k] : Inport  Port=4  SampleTime=pInitialization.Ts
  C[k] : Inport  Port=5  SampleTime=pInitialization.Ts
  D (unused) : Inport  Port=6  SampleTime=pInitialization.Ts
  xhat[k|k-1] : Inport  Port=7  SampleTime=pInitialization.Ts
  Add : Sum
  Enabled Subsystem : Subsystem  TreatAsAtomicUnit=on
  Terminator : Terminator
  Terminator1 : Terminator
  xhat[k|k] : Outport  SampleTime=pInitialization.Ts  VectorParamsAs1DForOutWhenUnconnected=off
  wires:
  Add/1 -> xhat[k|k]/1
  u (unused)/1 -> Terminator1/1
  D (unused)/1 -> Terminator/1
  M[k]/1 -> Enabled Subsystem/1(M[k])
  C[k]/1 -> Enabled Subsystem/2(C[k])
  y[k]/1 -> Enabled Subsystem/3(y[k])
  xhat[k|k-1]/1 -> Add/2, Enabled Subsystem/4(xhat[k|k-1])
  Enabled Subsystem/1(deltax) -> Add/1
  Enable[k]/1 -> Enabled Subsystem/Enable

== system softMBD_old/FCS/filters/Subsystem1/pitch_kalman/Kalman Filter1/checkA ==
  In1 : Inport
  u : Inport  Port=2
  Terminator : Terminator
  u_ : Outport  VectorParamsAs1DForOutWhenUnconnected=off
  wires:
  In1/1 -> Terminator/1
  u/1 -> u_/1

== system softMBD_old/FCS/filters/Subsystem1/pitch_kalman/Kalman Filter1/checkB ==
  In1 : Inport
  u : Inport  Port=2
  Terminator : Terminator
  u_ : Outport  VectorParamsAs1DForOutWhenUnconnected=off
  wires:
  In1/1 -> Terminator/1
  u/1 -> u_/1

== system softMBD_old/FCS/filters/Subsystem1/pitch_kalman/Kalman Filter1/checkC ==
  In1 : Inport
  u : Inport  Port=2
  Terminator : Terminator
  u_ : Outport  VectorParamsAs1DForOutWhenUnconnected=off
  wires:
  In1/1 -> Terminator/1
  u/1 -> u_/1

== system softMBD_old/FCS/filters/Subsystem1/pitch_kalman/Kalman Filter1/checkD ==
  In1 : Inport
  u : Inport  Port=2
  Terminator : Terminator
  u_ : Outport  VectorParamsAs1DForOutWhenUnconnected=off
  wires:
  In1/1 -> Terminator/1
  u/1 -> u_/1

== system softMBD_old/FCS/filters/Subsystem1/pitch_kalman/Kalman Filter1/checkEnable ==
  In1 : Inport
  u : Inport  Port=2
  Terminator : Terminator
  u_ : Outport  VectorParamsAs1DForOutWhenUnconnected=off
  wires:
  In1/1 -> Terminator/1
  u/1 -> u_/1

== system softMBD_old/FCS/filters/Subsystem1/pitch_kalman/Kalman Filter1/checkG ==
  In1 : Inport
  u : Inport  Port=2
  Terminator : Terminator
  u_ : Outport  VectorParamsAs1DForOutWhenUnconnected=off
  wires:
  In1/1 -> Terminator/1
  u/1 -> u_/1

== system softMBD_old/FCS/filters/Subsystem1/pitch_kalman/Kalman Filter1/checkH ==
  In1 : Inport
  u : Inport  Port=2
  Terminator : Terminator
  u_ : Outport  VectorParamsAs1DForOutWhenUnconnected=off
  wires:
  In1/1 -> Terminator/1
  u/1 -> u_/1

== system softMBD_old/FCS/filters/Subsystem1/pitch_kalman/Kalman Filter1/checkN ==
  In1 : Inport
  u : Inport  Port=2
  Terminator : Terminator
  u_ : Outport  VectorParamsAs1DForOutWhenUnconnected=off
  wires:
  In1/1 -> Terminator/1
  u/1 -> u_/1

== system softMBD_old/FCS/filters/Subsystem1/pitch_kalman/Kalman Filter1/checkP0 ==
  In1 : Inport
  u : Inport  Port=2
  Terminator : Terminator
  u_ : Outport  VectorParamsAs1DForOutWhenUnconnected=off
  wires:
  In1/1 -> Terminator/1
  u/1 -> u_/1

== system softMBD_old/FCS/filters/Subsystem1/pitch_kalman/Kalman Filter1/checkQ ==
  In1 : Inport
  u : Inport  Port=2
  Terminator : Terminator
  u_ : Outport  VectorParamsAs1DForOutWhenUnconnected=off
  wires:
  In1/1 -> Terminator/1
  u/1 -> u_/1

== system softMBD_old/FCS/filters/Subsystem1/pitch_kalman/Kalman Filter1/checkR ==
  In1 : Inport
  u : Inport  Port=2
  Terminator : Terminator
  u_ : Outport  VectorParamsAs1DForOutWhenUnconnected=off
  wires:
  In1/1 -> Terminator/1
  u/1 -> u_/1

== system softMBD_old/FCS/filters/Subsystem1/pitch_kalman/Kalman Filter1/checkReset ==
  In1 : Inport
  u : Inport  Port=2
  Terminator : Terminator
  u_ : Outport  VectorParamsAs1DForOutWhenUnconnected=off
  wires:
  In1/1 -> Terminator/1
  u/1 -> u_/1

== system softMBD_old/FCS/filters/Subsystem1/pitch_kalman/Kalman Filter1/checkX0 ==
  In1 : Inport
  u : Inport  Port=2
  Terminator : Terminator
  u_ : Outport  VectorParamsAs1DForOutWhenUnconnected=off
  wires:
  In1/1 -> Terminator/1
  u/1 -> u_/1

== system softMBD_old/FCS/filters/Subsystem1/pitch_kalman/Kalman Filter1/checku ==
  Ref : Inport
  u : Inport  Port=2
  CheckSignalProperties : S-Function  FunctionName=ctrlKalmanFilterCheckSignals  Parameters=parentBlockPath,portName,isContinuousTime,pInitialization.Ts,Ns,Nu,Nw,Ny  SFunctionDeploymentMode=off  EnableBusSupport=off
  y : Outport  VectorParamsAs1DForOutWhenUnconnected=off
  wires:
  u/1 -> CheckSignalProperties/2, y/1
  Ref/1 -> CheckSignalProperties/1

== system softMBD_old/FCS/filters/Subsystem1/pitch_kalman/Kalman Filter1/checky ==
  Ref : Inport
  u : Inport  Port=2
  CheckSignalProperties : S-Function  FunctionName=ctrlKalmanFilterCheckSignals  Parameters=parentBlockPath,portName,isContinuousTime,pInitialization.Ts,Ns,Nu,Nw,Ny  SFunctionDeploymentMode=off  EnableBusSupport=off
  y : Outport  VectorParamsAs1DForOutWhenUnconnected=off
  wires:
  u/1 -> CheckSignalProperties/2, y/1
  Ref/1 -> CheckSignalProperties/1
